simulink model "refrigerationCycle"  (R2014a)
settings: Solver=ode15s  StartTime=0.0  StopTime=3000  MaxStep=0.2  RelTol=1e-3  AbsTol=1e-3
PreLoadFcn:
  | load R134aProperties p_TLU u_TLU v_TLU T_TLU mu_TLU k_TLU Pr_TLU u_sat
  | 
  | % Refrigerant:
  | charge_pressure = 0.6; % MPa
  | initial_quality = 0.2;
  | 
  | % Environment:
  | environment_temperature = 293; % K
  | natural_convection_coefficient = 20; % W/m^2/K
  | 
  | % Controller:
  | target_temperature = 277; % K
  | temperature_delta = 2; % K
  | 
  | % Compressor:
  | commanded_mass_flow = 0.004; % kg/s
  | compressor_time_constant = 20; % s
  | 
  | % Expansion valve:
  | min_throat_area = 0.1; % mm^2
  | max_throat_area = 2.7; % mm^2
  | min_throat_temperature = 280; % K
  | max_throat_temperature = 230; % K
  | 
  | % Heat exchangers:
  | condenser_length = 15; % m
  | evaporator_length = 15; % m
  | fin_area = 1; % m^2
  | fin_convection_coefficient = 150; % W/m^2/K
  | 
  | % Pipes:
  | pipe_diameter = 0.015; % m
  | pipe_thickness = 0.0005; % m
  | 
  | % Refrigerator compartment:
  | interior_surface_area = 4.5; % m^2
  | exterior_surface_area = 6; % m^2
  | foam_thickness = 0.03; % m
  | 
  | % Material properties:
  | copper_density = 8940; % kg/m^3
  | copper_specific_heat = 390; % J/kg/K
  | copper_conductivity = 400; % W/m/K
  | foam_conductivity = 0.03; % W/m/K
undefined symbols (not defined in the file or in its folder): u_sat
libraries: fl_lib x25, refrigeration_lib x19, nesl_utility x5
Description:
  | Two-Phase Flow Refrigeration Model
  | 
  | This example demonstrates a two-phase flow model to simulate a refrigeration cycle.
  | The compressor drives the R-134a refrigerant through a condenser, an expansion valve,
  | and an evaporator. The hot gas leaving the compressor condenses in the condenser via
  | heat transfer to the environment. The pressure drops as the refrigerant passes through
  | the expansion valve. The drop in pressure causes the refrigerant to boil in the evaporator
  | as it absorbs heat from the refrigerator compartment. The refrigeration then returns to
  | the compressor to repeat the cycle. The controller turns the compressor on and off to
  | maintain the refrigerator compartment temperature within a band around the desired
  | temperature.
  | 
  | Copyright 2013-2014 The MathWorks, Inc.
settings Model: Creator=MathWorks  LastModifiedBy=leong
settings SolverCC: MaxConsecutiveMinStep=2
settings DataIOCC: LimitDataPoints=off  SignalLoggingSaveFormat=ModelDataLogs
settings DebuggingCC: MergeDetectMultiDrivingBlocksExec=error  MultiTaskDSMMsg=warning  MultiTaskCondExecSysMsg=none
settings RTWCC: IncludeERTFirstTime=on
settings SimscapeCC: SimscapeLogType=all  SimscapeLogName=refrigerationModelData  SimscapeLogLimitData=off

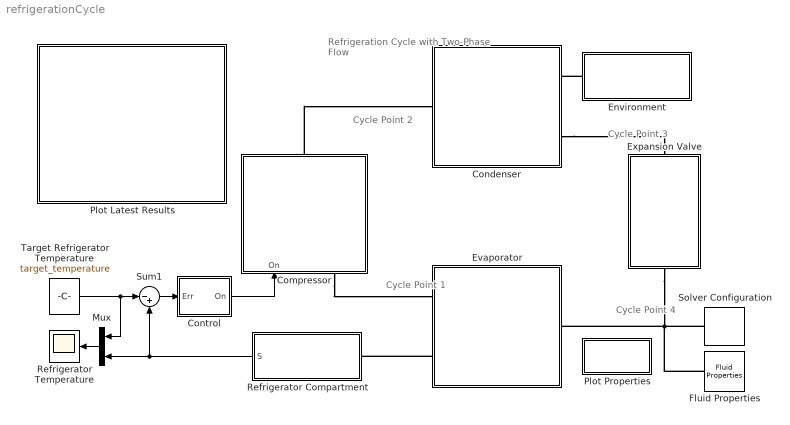
== system refrigerationCycle ==
  note: Cycle Point 1
  note: Cycle Point 2
  note: Cycle Point 3
  note: Refrigeration Cycle
      | with Two-Phase Flow
  note: Cycle Point 4
  Compressor : Subsystem
      mask Display:
      | % Fading color
      | % Center to right
      | patch(sin(0.00*pi:0.05:1.10*pi),cos(0.00*pi:0.05:1.10*pi),[1;0.90;0.94]);
      | patch(sin(0.05*pi:0.05:0.95*pi),cos(0.05*pi:0.05:0.95*pi),[1;0.85;0.88]);
      | patch(sin(0.10*pi:0.05:0.90*pi),cos(0.10*pi:0.05:0.90*pi),[1;0.80;0.82]);
      | patch(sin(0.15*pi:0.05:0.85*pi),cos(0.15*pi:0.05:0.85*pi),[1;0.75;0.76]);
      | patch(sin(0.20*pi:0.05:0.80*pi),cos(0.20*pi:0.05:0.80*pi),[1;0.70;0.70]);
      | % Center to left
      | patch(sin(1.00*pi:0.05:2.00*pi),cos(1.00*pi:0.05:2.00*pi),[0.94;0.90;1]);
      | patch(sin(1.05*pi:0.05:1.95*pi),cos(1.05*pi:0.05:1.95*pi),[0.88;0.90;1]);
      | patch(sin(1.10*pi:0.05:1.90*pi),cos(1.10*pi:0.05:1.90*pi),[0.82;0.90;1]);
      | patch(sin(1.15*pi:0.05:1.85*pi),cos(1.15*pi:0.05:1.85*pi),[0.76;0.90;1]);
      | patch(sin(1.20*pi:0.05:1.80*pi),cos(1.20*pi:0.05:1.80*pi),[0.70;0.90;1]);
      | % Circle
      | plot(sin(0:0.1:2.2*pi),cos(0:0.1:2.2*pi));
      | % Angled lines
      | plot(sin([-0.6*pi/3 3.6*pi/8]),cos([-0.6*pi/3 3.6*pi/8]));
      | plot(sin([-0.6*pi/3 3.6*pi/8]),-cos([-0.6*pi/3 3.6*pi/8]));
      | plot(1.15*sin([-pi/4 3*pi/4]),1.15*cos([-pi/4 3*pi/4]));
      | % Arrow
      | patch([1.15*sin(-pi/4)+0.01;1.15*sin(3*pi/4)+0.01;1.15*sin(3*pi/4)-0.01;1.15*sin(-pi/4)-0.01],[1.15*cos(-pi/4)+0.01;1.15*cos(3*pi/4)+0.01;1.15*cos(3*pi/4)-0.01;1.15*cos(-pi/4)-0.01],[0;0;0])
      | patch([0.8*sin(3*pi/4)+0.05;1.15*sin(3*pi/4)+0.00;1.15*sin(3*pi/4)-0.00;0.8*sin(3*pi/4)-0.05],[0.8*cos(3*pi/4)+0.05;1.15*cos(3*pi/4)+0.00;1.15*cos(3*pi/4)-0.00;0.8*cos(3*pi/4)-0.05],[0;0;0])
      | % Points to set range for plotting area
      | color('white');plot(1.3,1.3);plot(-1.3,-1.3)
      | color('black');
      | 
      | port_label('LConn',1,'A');
      | port_label('RConn',1,'B');
      | port_label('input',1,'On');
  Condenser : Subsystem
      mask Display:
      | % Colored patches
      | % Center to right
      | patch(sin(0.0*pi:0.05:1.1*pi),cos(0.0*pi:0.05:1.1*pi),[1;0.58;0.58]);
      | patch(sin(0.1*pi:0.05:0.9*pi),cos(0.1*pi:0.05:0.9*pi),[1;0.64;0.64]);
      | patch(sin(0.2*pi:0.05:0.8*pi),cos(0.2*pi:0.05:0.8*pi),[1;0.70;0.70]);
      | % Center to left
      | patch(sin(1.0*pi:0.05:2.0*pi),cos(1.0*pi:0.05:2.0*pi),[1;0.52;0.52]);
      | patch(sin(1.1*pi:0.05:1.9*pi),cos(1.1*pi:0.05:1.9*pi),[1;0.46;0.46]);
      | patch(sin(1.2*pi:0.05:1.8*pi),cos(1.2*pi:0.05:1.8*pi),[1;0.40;0.40]);
      | % Circle
      | plot(sin(0:0.1:2.2*pi),cos(0:0.1:2.2*pi));
      | % 'M'
      | plot([0.5 0.5],[-1.2 0.5]);
      | plot([-0.5 -0.5],[-1.2 0.5]);
      | plot([0.5 0],[0.5 -0.2]);
      | plot([-0.5 0],[0.5 -0.2]);
      | % Plot points to set plot range
      | color('white');plot(1.3,1.3);plot(-1.3,-1.3)
      | color('black');
      | 
      | port_label('RConn',1,'A');
      | port_label('LConn',1,'T');
      | port_label('LConn',2,'B');
  Control : Subsystem
  Environment : Subsystem
      mask Display:
      | % Colored patch
      | patch([sin(0:0.1:1*pi)*0.25+0.4 sin(pi:0.1:2*pi)*0.25-0.4],[cos(0:0.1:1*pi) cos(pi:0.1:2*pi)],[1;0.9;0.9]);
      | % Outer rounded rectangle
      | plot(sin(0:0.1:1*pi)*0.25+0.4,cos(0:0.1:1*pi));
      | plot(sin(pi:0.1:2*pi)*0.25-0.4,cos(pi:0.1:2*pi));
      | plot([-0.4 0.4],[1 1]);
      | plot([-0.4 0.4],[-1 -1]);
      | % House frame
      | plot([-0.3 -0.3],[-0.866,0.866*0.2])
      | plot([0.3 0.3],[-0.866,0.866*0.2])
      | plot([0.3 0],[0.866*0.2, 0.866])
      | plot([-0.3 0],[0.866*0.2, 0.866])
      | plot([-0.3 0.3],[-0.866 -0.866])
      | plot([-0.3 0.3],[0.866 0.866]*0.2)
      | plot([-0.2 -0.04],[0.866 0.866]*0)
      | % Window
      | plot([-0.2 -0.04],[-1 -1]*0.2)
      | plot([-0.2 -0.04],[-1 -1]*0.4)
      | plot([-0.2 -0.2],[0 -0.4])
      | plot([-0.12 -0.12],[0 -0.4])
      | plot([-0.04 -0.04],[0 -0.4])
      | % Door
      | plot([0.05 0.05],[-0.866 -0.2])
      | plot([0.18 0.18],[-0.866 -0.2])
      | plot([0.05 0.18],[-0.2 -0.2])
      | patch([0.12 0.15 0.12 0.15],[-0.5 -0.5 -0.54 -0.54],[0;0;0])
      | % Outer boundary (so plot labels are visible)
      | color('white');plot(0.8660,0.8660);plot(-0.8660,-0.8660)
      | color('black');
      | port_label('LConn',1,'T');
  Evaporator : Subsystem
      mask Display:
      | % Fading color
      | % Center to right
      | patch(sin(0.00*pi:0.05:1.10*pi),cos(0.00*pi:0.05:1.10*pi),[0.58;0.70;1]);
      | patch(sin(0.05*pi:0.05:0.95*pi),cos(0.05*pi:0.05:0.95*pi),[0.63;0.75;1]);
      | patch(sin(0.10*pi:0.05:0.90*pi),cos(0.10*pi:0.05:0.90*pi),[0.66;0.80;1]);
      | patch(sin(0.15*pi:0.05:0.85*pi),cos(0.15*pi:0.05:0.85*pi),[0.69;0.85;1]);
      | patch(sin(0.20*pi:0.05:0.80*pi),cos(0.20*pi:0.05:0.80*pi),[0.70;0.90;1]);
      | % Center to left
      | patch(sin(1.00*pi:0.05:2.00*pi),cos(1.00*pi:0.05:2.00*pi),[0.52;0.60;1]);
      | patch(sin(1.05*pi:0.05:1.95*pi),cos(1.05*pi:0.05:1.95*pi),[0.49;0.55;1]);
      | patch(sin(1.10*pi:0.05:1.90*pi),cos(1.10*pi:0.05:1.90*pi),[0.46;0.50;1]);
      | patch(sin(1.15*pi:0.05:1.85*pi),cos(1.15*pi:0.05:1.85*pi),[0.43;0.45;1]);
      | patch(sin(1.20*pi:0.05:1.80*pi),cos(1.20*pi:0.05:1.80*pi),[0.40;0.40;1]);
      | % Circle
      | plot(sin(0:0.1:2.2*pi),cos(0:0.1:2.2*pi));
      | % 'M'
      | plot([0.5 0.5],[-1.2 0.5]);
      | plot([-0.5 -0.5],[-1.2 0.5]);
      | plot([0.5 0],[0.5 -0.2]);
      | plot([-0.5 0],[0.5 -0.2]);
      | % Plot points to set plotting range
      | color('white');plot(1.3,1.3);plot(-1.3,-1.3)
      | color('black');
      | 
      | port_label('LConn',1,'A');
      | port_label('RConn',1,'B');
      | port_label('RConn',2,'T');
  Expansion Valve : Subsystem
      mask Display:
      | % Colored patches
      | patch([-1 -1 0],[0.5 -0.5 0],[1;0.4;0.4]);
      | patch([1 1 0],[0.5 -0.5 0],[0.4;0.4;1]);
      | % Valve
      | plot([1 1],[0.5 -0.5]);
      | plot([-1 -1],[0.5 -0.5]);
      | plot([-1 1],[0.5 -0.5]);
      | plot([-1 1],[-0.5 0.5]);
      | % Arrow
      | patch([1.15*sin(-pi/4-0.01);1.15*sin(-pi/4+0.01);1*sin(3*pi/4-0.01);1*sin(3*pi/4+0.01)],[1.15*cos(-pi/4-0.01);1.15*cos(-pi/4+0.01);1*cos(3*pi/4-0.01);1*cos(3*pi/4+0.01)],[0;0;0])
      | patch([0.8*sin(3*pi/4+0.07);1.15*sin(3*pi/4+0.00);1.15*sin(3*pi/4-0.00);0.8*sin(3*pi/4-0.07)],[0.8*cos(3*pi/4+0.07);1.15*cos(3*pi/4+0.00);1.15*cos(3*pi/4-0.00);0.8*cos(3*pi/4-0.07)],[0;0;0])
      | % Plot outer points to set plot range
      | color('white'); plot(-1.3,0); plot(1.3,0);
      | color('black');
      | port_label('LConn',1,'A');
      | port_label('RConn',1,'B');
  Fluid Properties : refrigeration_lib/Fluid Properties  p_TLU=p_TLU MPa  u_TLU=u_TLU kJ/kg  v_TLU=v_TLU m^3/kg  T_TLU=T_TLU K  mu_TLU=mu_TLU s*uPa  k_TLU=k_TLU W/(m*K)  Pr_TLU=Pr_TLU  u_liq=u_sat(:,1) kJ/kg  u_vap=u_sat(:,2) kJ/kg
  Mux : Mux  Inputs=2
  Plot Latest Results : Subsystem
      settings: OpenFcn=|
      | if exist('refrigerationModelData')
      |    plotRefrigerationModel(refrigerationModelData);
      | else
      |    errordlg('Simulate refrigerationCycle.slx before plotting results');
      | end
      mask Display: image('phDiagram.png')
  Plot Properties : Subsystem
      settings: OpenFcn=plotFluidProperties()
      mask Display: disp('Plot Fluid\nProperties');
  Refrigerator Compartment : Subsystem
      mask Display:
      | % Color
      | patch([sin(0:0.1:1*pi)*0.25+0.4 sin(pi:0.1:2*pi)*0.25-0.4],[cos(0:0.1:1*pi) cos(pi:0.1:2*pi)],[0.70;0.90;1]);
      | % Outer rounded rectangle
      | plot(sin(pi:0.1:2*pi)*0.25-0.4,cos(pi:0.1:2*pi));
      | plot(sin(0:0.1:1*pi)*0.25+0.4,cos(0:0.1:1*pi));
      | plot(sin(pi:0.1:2*pi)*0.25-0.4,cos(pi:0.1:2*pi));
      | plot([-0.4 0.4],[1 1]);
      | plot([-0.4 0.4],[-1 -1]);
      | % Outer points to set size of plot range
      | color('white');plot(0.8660,0.8660);plot(-0.8660,-0.8660)
      | color('black');
      | % Snowflake
      | plot([0 0],[0.8 -0.8]);
      | plot([0 0.1],[0.5 0.7]);
      | plot([0 -0.1],[0.5 0.7]);
      | plot([0 0.1],[-0.5 -0.7]);
      | plot([0 -0.1],[-0.5 -0.7]);
      | plot(0.3*sin([pi/3 4*pi/3]),1*cos([pi/3 4*pi/3]));
      | plot([0.22*sin(pi/3) 0.25*sin(pi/4)],[0.7*cos(pi/3) 0.84*cos(pi/4)]);
      | plot([0.22*sin(pi/3) 0.25*sin(pi/2)],[0.7*cos(pi/3) 0.325*cos(pi/4)]);
      | plot([0.22*sin(pi/3) 0.25*sin(pi/4)],[-0.7*cos(pi/3) -0.84*cos(pi/4)]);
      | plot([0.22*sin(pi/3) 0.25*sin(pi/2)],[-0.7*cos(pi/3) -0.325*cos(pi/4)]);
      | plot(-0.3*sin([pi/3 4*pi/3]),1*cos([pi/3 4*pi/3]));
      | plot([-0.22*sin(pi/3) -0.25*sin(pi/4)],[0.7*cos(pi/3) 0.84*cos(pi/4)]);
      | plot([-0.22*sin(pi/3) -0.25*sin(pi/2)],[0.7*cos(pi/3) 0.325*cos(pi/4)]);
      | plot([-0.22*sin(pi/3) -0.25*sin(pi/4)],[-0.7*cos(pi/3) -0.84*cos(pi/4)]);
      | plot([-0.22*sin(pi/3) -0.25*sin(pi/2)],[-0.7*cos(pi/3) -0.325*cos(pi/4)]);
      | plot([0 0.1],[-0.5 -0.7]);
      | plot([0 -0.1],[-0.5 -0.7]);
      | % Labels
      | port_label('LConn',1,'T');
      | port_label('output',1,'S');
  Refrigerator Temperature : Scope
      settings: TimeRange=3000  YMin=274  YMax=280  SaveName=T
  Solver Configuration : nesl_utility/Solver Configuration  PhysicalDomain=network_engine_domain  SubClassName=solver  LeftPortType=input  RightPortType=generic  Accelerate=off  Tones=[]  Harmonics=[]  SimulateNoise=off  Profile=off  UseLocalSampling=off  EnableSwitchedLinearOptims=on  FrequencyDomain=off  UseCCode=off  RelTol=0.001  AbsTol=1e-06  MinStep=1e-09  ToWorkspace=off  DoDC=off  ResidualTolerance=1e-9  UseLocalSolver=off  LocalSolverChoice=NE_TRAPEZOIDAL_ADVANCER  LocalSolverSampleTime=0.1  DoFixedCost=off  MaxNonlinIter=3  MaxModeIter=2  LinearAlgebra=Sparse  DelaysMemoryBudget=1024  AutomaticFiltering=on  FilteringTimeConstant=0.001
  Sum1 : Sum  Inputs=|-+
  Target Refrigerator Temperature : Constant  Value=target_temperature
  wires:
  Target Refrigerator Temperature/1 -> Sum1/1, Mux/1
  Refrigerator Compartment/1(S) -> Mux/2, Sum1/2
  Sum1/1 -> Control/1(Err)
  Control/1(On) -> Compressor/1(On)
  Mux/1 -> Refrigerator Temperature/1
  connections:
  Solver Configuration/RConn1 -- Fluid Properties/RConn1 -- Evaporator/LConn1 -- Expansion Valve/RConn1
  Compressor/RConn1 -- Condenser/RConn1
  Evaporator/RConn2 -- Refrigerator Compartment/LConn1
  Compressor/LConn1 -- Evaporator/RConn1
  Environment/LConn1 -- Condenser/LConn1
  Condenser/LConn2 -- Expansion Valve/LConn1

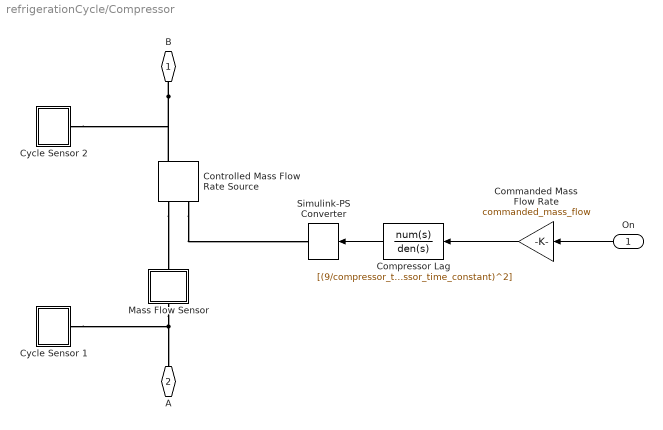
== system refrigerationCycle/Compressor ==
  On : Inport
  Commanded Mass Flow Rate : Gain  Gain=commanded_mass_flow
  Compressor Lag : TransferFcn  Numerator=[(9/compressor_time_constant)^2]  Denominator=[1, 2*(9/compressor_time_constant), (9/compressor_time_constant)^2]
  Controlled Mass Flow Rate Source : refrigeration_lib/Controlled Mass Flow Rate Source  S=pi*pipe_diameter^2/4 m^2  L=0.1 m  mdot_specify=off  mdot_priority=High  mdot=0 kg/s  phi_A_specify=off  phi_A_priority=High  phi_A=0 kW  phi_B_specify=off  phi_B_priority=High  phi_B=0 kW  u_AI_specify=off  u_AI_priority=High  u_AI=396.921741345 kJ/kg  v_A_specify=off  v_A_priority=High  v_A=0.230606289431 m^3/kg  u_BI_specify=off  u_BI_priority=High  u_BI=396.921741345 kJ/kg  v_B_specify=off  v_B_priority=High  v_B=0.230606289431 m^3/kg  u_2_specify=off  u_2_priority=High  u_2=396.921741345 kJ/kg  u_3_specify=off  u_3_priority=High  u_3=396.921741345 kJ/kg
  Cycle Sensor 1 : Subsystem
  Cycle Sensor 2 : Subsystem
  Mass Flow Sensor : Subsystem
  Simulink-PS Converter : nesl_utility/Simulink-PS Converter  PhysicalDomain=network_engine_domain  SubClassName=ps_input  LeftPortType=input  RightPortType=output  PseudoPeriodic=off  Frequencies=[]  NoiseDistribution=none  NoiseParameters=[]  Unit=kg/s  AffineConversion=off  InputFiltering=off  SimscapeFilterOrder=1  InputFilterTimeConstant=0.001  UdotUserProvided=1
  B : PMIOPort  Port=1  Side=Right
  A : PMIOPort  Port=2  Side=Left
  wires:
  Compressor Lag/1 -> Simulink-PS Converter/1
  Commanded Mass Flow Rate/1 -> Compressor Lag/1
  On/1 -> Commanded Mass Flow Rate/1
  connections:
  B/RConn1 -- Cycle Sensor 2/LConn1 -- Controlled Mass Flow Rate Source/RConn1
  Controlled Mass Flow Rate Source/LConn2 -- Simulink-PS Converter/RConn1
  Controlled Mass Flow Rate Source/LConn1 -- Mass Flow Sensor/RConn1
  Mass Flow Sensor/LConn1 -- A/RConn1 -- Cycle Sensor 1/LConn1

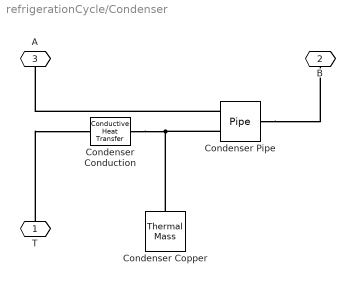
== system refrigerationCycle/Condenser ==
  Condenser Conduction : fl_lib/Thermal/Thermal Elements/Conductive Heat Transfer  area=pi*pipe_diameter*condenser_length m^2  thickness=pipe_thickness m  th_cond=copper_conductivity W/(m*K)  Q_specify=off  Q_priority=High  Q=0 J/s  T_specify=off  T_priority=High  T=0 K
  Condenser Copper : fl_lib/Thermal/Thermal Elements/Thermal Mass  mass=pi*pipe_diameter*condenser_length*pipe_thickness*copper_density kg  sp_heat=copper_specific_heat J/kg/K  Q_specify=off  Q_priority=High  Q=0 J/s  T_specify=on  T_priority=High  T=environment_temperature K
  Condenser Pipe : refrigeration_lib/Pipe  L=condenser_length m  S=pi*pipe_diameter^2/4 m^2  Dh=pipe_diameter m  fs=64  La=0.1*condenser_length m  eps=15e-6 m  Re_lam=2000  Re_tur=4000  J_smooth=5 kg/m^2/s  p_0=charge_pressure MPa  T_0=-1 K  x_0=initial_quality  mdot_A_specify=off  mdot_A_priority=High  mdot_A=0 kg/s  mdot_B_specify=off  mdot_B_priority=High  mdot_B=0 kg/s  phi_A_specify=off  phi_A_priority=High  phi_A=0 kW  phi_B_specify=off  phi_B_priority=High  phi_B=0 kW  v_A_specify=off  v_A_priority=High  v_A=0.230606289431 m^3/kg  v_B_specify=off  v_B_priority=High  v_B=0.230606289431 m^3/kg  p_I_specify=off  p_I_priority=High  p_I=0.101325 MPa  u_I_specify=off  u_I_priority=High  u_I=396.921741345 kJ/kg  v_I_specify=off  v_I_priority=High  v_I=0.230606289431 m^3/kg  q_T_specify=off  q_T_priority=High  q_T=0 kW  Ff_A_specify=off  Ff_A_priority=High  Ff_A=0 N  Ff_B_specify=off  Ff_B_priority=High  Ff_B=0 N  ev_I_specify=off  ev_I_priority=High  ev_I=1.7212095226213e+3 kJ/m^3  mdot_I_specify=off  mdot_I_priority=High  mdot_I=0 kg/s  Nu_I_specify=off  Nu_I_priority=High  Nu_I=0
  T : PMIOPort  Port=1  Side=Left
  B : PMIOPort  Port=2  Side=Left
  A : PMIOPort  Port=3  Side=Right
  connections:
  Condenser Pipe/LConn1 -- A/RConn1
  Condenser Conduction/LConn1 -- Condenser Pipe/LConn2 -- Condenser Copper/LConn1
  T/RConn1 -- Condenser Conduction/RConn1
  Condenser Pipe/RConn1 -- B/RConn1

== system refrigerationCycle/Control ==
  Err : Inport
  Relay : Relay  OnSwitchValue=temperature_delta  OffSwitchValue=-temperature_delta
  On : Outport
  wires:
  Err/1 -> Relay/1
  Relay/1 -> On/1

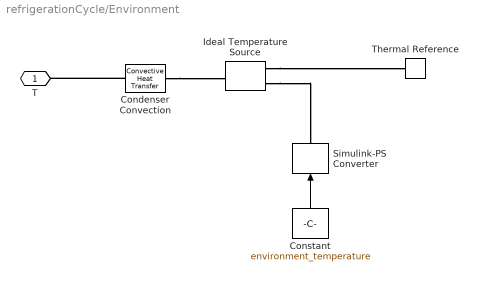
== system refrigerationCycle/Environment ==
  Condenser Convection : fl_lib/Thermal/Thermal Elements/Convective Heat Transfer  area=fin_area m^2  heat_tr_coeff=fin_convection_coefficient W/(m^2 * K)  Q_specify=off  Q_priority=High  Q=0 J/s  T_specify=off  T_priority=High  T=0 K
  Constant : Constant  Value=environment_temperature
  Ideal Temperature Source : fl_lib/Thermal/Thermal Sources/Ideal Temperature Source
  Simulink-PS Converter : nesl_utility/Simulink-PS Converter  PhysicalDomain=network_engine_domain  SubClassName=ps_input  LeftPortType=input  RightPortType=output  PseudoPeriodic=off  Frequencies=[]  NoiseDistribution=none  NoiseParameters=[]  Unit=K  AffineConversion=off  InputFiltering=off  SimscapeFilterOrder=1  InputFilterTimeConstant=0.001  UdotUserProvided=1
  Thermal Reference : fl_lib/Thermal/Thermal Elements/Thermal Reference
  T : PMIOPort  Port=1  Side=Left
  wires:
  Constant/1 -> Simulink-PS Converter/1
  connections:
  Condenser Convection/RConn1 -- Ideal Temperature Source/LConn1
  Condenser Convection/LConn1 -- T/RConn1
  Ideal Temperature Source/RConn1 -- Simulink-PS Converter/RConn1
  Ideal Temperature Source/RConn2 -- Thermal Reference/LConn1

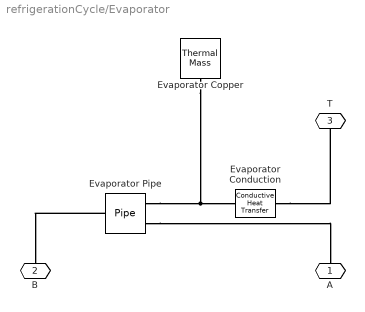
== system refrigerationCycle/Evaporator ==
  Evaporator Conduction : fl_lib/Thermal/Thermal Elements/Conductive Heat Transfer  area=pi*pipe_diameter*evaporator_length m^2  thickness=pipe_thickness m  th_cond=copper_conductivity W/(m*K)  Q_specify=off  Q_priority=High  Q=0 J/s  T_specify=off  T_priority=High  T=0 K
  Evaporator Copper : fl_lib/Thermal/Thermal Elements/Thermal Mass  mass=pi*pipe_diameter*evaporator_length*pipe_thickness*copper_density kg  sp_heat=copper_specific_heat J/kg/K  Q_specify=off  Q_priority=High  Q=0 J/s  T_specify=on  T_priority=High  T=target_temperature K
  Evaporator Pipe : refrigeration_lib/Pipe  L=evaporator_length m  S=pi*pipe_diameter^2/4 m^2  Dh=pipe_diameter m  fs=64  La=0.1*evaporator_length m  eps=15e-6 m  Re_lam=2000  Re_tur=4000  J_smooth=5 kg/m^2/s  p_0=charge_pressure MPa  T_0=-1 K  x_0=initial_quality  mdot_A_specify=off  mdot_A_priority=High  mdot_A=0 kg/s  mdot_B_specify=off  mdot_B_priority=High  mdot_B=0 kg/s  phi_A_specify=off  phi_A_priority=High  phi_A=0 kW  phi_B_specify=off  phi_B_priority=High  phi_B=0 kW  v_A_specify=off  v_A_priority=High  v_A=0.230606289431 m^3/kg  v_B_specify=off  v_B_priority=High  v_B=0.230606289431 m^3/kg  p_I_specify=off  p_I_priority=High  p_I=0.101325 MPa  u_I_specify=off  u_I_priority=High  u_I=396.921741345 kJ/kg  v_I_specify=off  v_I_priority=High  v_I=0.230606289431 m^3/kg  q_T_specify=off  q_T_priority=High  q_T=0 kW  Ff_A_specify=off  Ff_A_priority=High  Ff_A=0 N  Ff_B_specify=off  Ff_B_priority=High  Ff_B=0 N  ev_I_specify=off  ev_I_priority=High  ev_I=1.7212095226213e+3 kJ/m^3  mdot_I_specify=off  mdot_I_priority=High  mdot_I=0 kg/s  Nu_I_specify=off  Nu_I_priority=High  Nu_I=0
  A : PMIOPort  Port=1  Side=Left
  B : PMIOPort  Port=2  Side=Right
  T : PMIOPort  Port=3  Side=Right
  connections:
  Evaporator Conduction/RConn1 -- T/RConn1
  Evaporator Copper/LConn1 -- Evaporator Pipe/LConn2 -- Evaporator Conduction/LConn1
  Evaporator Pipe/RConn1 -- B/RConn1
  Evaporator Pipe/LConn1 -- A/RConn1

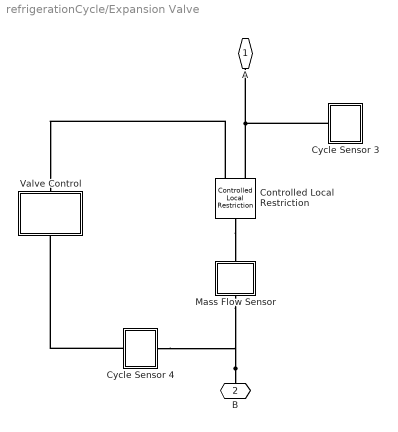
== system refrigerationCycle/Expansion Valve ==
  Controlled Local Restriction : refrigeration_lib/Controlled Local Restriction  Cd=0.7  L=0.1 m  S=pi*pipe_diameter^2/4 m^2
  Cycle Sensor 3 : Subsystem
  Cycle Sensor 4 : Subsystem
  Mass Flow Sensor : Subsystem
  Valve Control : Subsystem
  A : PMIOPort  Port=1  Side=Left
  B : PMIOPort  Port=2  Side=Right
  connections:
  B/RConn1 -- Cycle Sensor 4/LConn1 -- Mass Flow Sensor/RConn1
  Cycle Sensor 3/LConn1 -- Controlled Local Restriction/LConn1 -- A/RConn1
  Controlled Local Restriction/RConn1 -- Mass Flow Sensor/LConn1
  Controlled Local Restriction/LConn2 -- Valve Control/LConn1
  Cycle Sensor 4/RConn1 -- Valve Control/RConn1

== system refrigerationCycle/Plot Latest Results ==

== system refrigerationCycle/Plot Properties ==

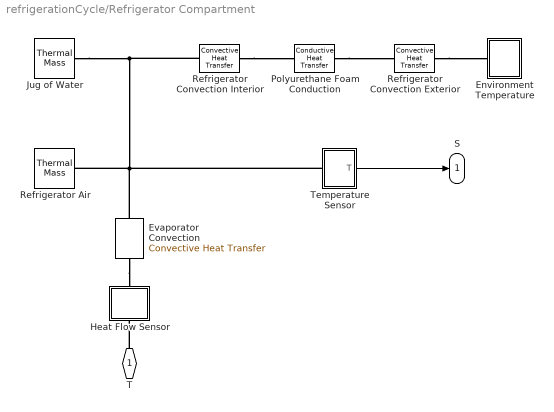
== system refrigerationCycle/Refrigerator Compartment ==
  Environment Temperature : Subsystem
  Evaporator Convection : fl_lib/Thermal/Thermal Elements/Convective Heat Transfer  area=interior_surface_area m^2  heat_tr_coeff=natural_convection_coefficient W/(m^2 * K)  Q_specify=off  Q_priority=High  Q=0 J/s  T_specify=off  T_priority=High  T=0 K
  Heat Flow Sensor : Subsystem
  Jug of Water : fl_lib/Thermal/Thermal Elements/Thermal Mass  mass=3.8 kg  sp_heat=4187 J/kg/K  Q_specify=off  Q_priority=High  Q=0 J/s  T_specify=on  T_priority=High  T=target_temperature K
  Polyurethane Foam Conduction : fl_lib/Thermal/Thermal Elements/Conductive Heat Transfer  area=interior_surface_area m^2  thickness=foam_thickness m  th_cond=foam_conductivity W/(m*K)  Q_specify=off  Q_priority=High  Q=0 J/s  T_specify=off  T_priority=High  T=0 K
  Refrigerator Air : fl_lib/Thermal/Thermal Elements/Thermal Mass  mass=1 kg  sp_heat=1012 J/kg/K  Q_specify=off  Q_priority=High  Q=0 J/s  T_specify=on  T_priority=High  T=target_temperature K
  Refrigerator Convection Exterior : fl_lib/Thermal/Thermal Elements/Convective Heat Transfer  area=exterior_surface_area m^2  heat_tr_coeff=natural_convection_coefficient W/(m^2 * K)  Q_specify=off  Q_priority=High  Q=0 J/s  T_specify=off  T_priority=High  T=0 K
  Refrigerator Convection Interior : fl_lib/Thermal/Thermal Elements/Convective Heat Transfer  area=interior_surface_area m^2  heat_tr_coeff=natural_convection_coefficient W/(m^2 * K)  Q_specify=off  Q_priority=High  Q=0 J/s  T_specify=off  T_priority=High  T=0 K
  Temperature Sensor : Subsystem
  T : PMIOPort  Port=1  Side=Left
  S : Outport
  wires:
  Temperature Sensor/1(T) -> S/1
  connections:
  Evaporator Convection/LConn1 -- Heat Flow Sensor/RConn1
  T/RConn1 -- Heat Flow Sensor/LConn1
  Refrigerator Convection Exterior/RConn1 -- Environment Temperature/LConn1
  Refrigerator Convection Interior/LConn1 -- Jug of Water/LConn1 -- Refrigerator Air/LConn1 -- Temperature Sensor/LConn1 -- Evaporator Convection/RConn1
  Refrigerator Convection Interior/RConn1 -- Polyurethane Foam Conduction/LConn1
  Polyurethane Foam Conduction/RConn1 -- Refrigerator Convection Exterior/LConn1

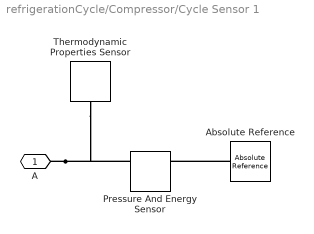
== system refrigerationCycle/Compressor/Cycle Sensor 1 ==
  Absolute Reference : refrigeration_lib/Absolute Reference  mdot_A_specify=off  mdot_A_priority=High  mdot_A=0 kg/s  phi_A_specify=off  phi_A_priority=High  phi_A=0 kW
  Pressure And Energy Sensor : refrigeration_lib/Pressure And Energy Sensor  mdot_specify=off  mdot_priority=High  mdot=0 kg/s  phi_specify=off  phi_priority=High  phi=0 kW
  Thermodynamic Properties Sensor : refrigeration_lib/Thermodynamic Properties Sensor  mdot_A_specify=off  mdot_A_priority=High  mdot_A=0 kg/s  phi_A_specify=off  phi_A_priority=High  phi_A=0 kW
  A : PMIOPort  Port=1  Side=Left
  connections:
  Absolute Reference/LConn1 -- Pressure And Energy Sensor/RConn1
  A/RConn1 -- Thermodynamic Properties Sensor/RConn1 -- Pressure And Energy Sensor/LConn1

== system refrigerationCycle/Compressor/Cycle Sensor 2 ==
  Absolute Reference : refrigeration_lib/Absolute Reference  mdot_A_specify=off  mdot_A_priority=High  mdot_A=0 kg/s  phi_A_specify=off  phi_A_priority=High  phi_A=0 kW
  Pressure And Energy Sensor : refrigeration_lib/Pressure And Energy Sensor  mdot_specify=off  mdot_priority=High  mdot=0 kg/s  phi_specify=off  phi_priority=High  phi=0 kW
  Thermodynamic Properties Sensor : refrigeration_lib/Thermodynamic Properties Sensor  mdot_A_specify=off  mdot_A_priority=High  mdot_A=0 kg/s  phi_A_specify=off  phi_A_priority=High  phi_A=0 kW
  A : PMIOPort  Port=1  Side=Left
  connections:
  Absolute Reference/LConn1 -- Pressure And Energy Sensor/RConn1
  Pressure And Energy Sensor/LConn1 -- A/RConn1 -- Thermodynamic Properties Sensor/RConn1

== system refrigerationCycle/Compressor/Mass Flow Sensor ==
  Mass And Energy Flow Sensor : refrigeration_lib/Mass And Energy Flow Sensor  mdot_specify=off  mdot_priority=High  mdot=0 kg/s  phi_specify=off  phi_priority=High  phi=0 kW
  B : PMIOPort  Port=1  Side=Right
  A : PMIOPort  Port=2  Side=Left
  connections:
  Mass And Energy Flow Sensor/RConn1 -- B/RConn1
  Mass And Energy Flow Sensor/LConn1 -- A/RConn1

== system refrigerationCycle/Expansion Valve/Cycle Sensor 3 ==
  Absolute Reference : refrigeration_lib/Absolute Reference  mdot_A_specify=off  mdot_A_priority=High  mdot_A=0 kg/s  phi_A_specify=off  phi_A_priority=High  phi_A=0 kW
  Pressure And Energy Sensor : refrigeration_lib/Pressure And Energy Sensor  mdot_specify=off  mdot_priority=High  mdot=0 kg/s  phi_specify=off  phi_priority=High  phi=0 kW
  Thermodynamic Properties Sensor : refrigeration_lib/Thermodynamic Properties Sensor  mdot_A_specify=off  mdot_A_priority=High  mdot_A=0 kg/s  phi_A_specify=off  phi_A_priority=High  phi_A=0 kW
  A : PMIOPort  Port=1  Side=Left
  connections:
  Absolute Reference/LConn1 -- Pressure And Energy Sensor/RConn1
  Pressure And Energy Sensor/LConn1 -- A/RConn1 -- Thermodynamic Properties Sensor/RConn1

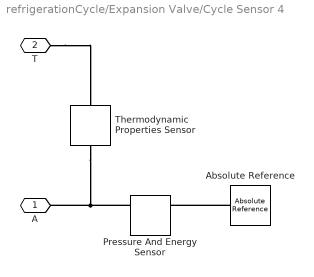
== system refrigerationCycle/Expansion Valve/Cycle Sensor 4 ==
  Absolute Reference : refrigeration_lib/Absolute Reference  mdot_A_specify=off  mdot_A_priority=High  mdot_A=0 kg/s  phi_A_specify=off  phi_A_priority=High  phi_A=0 kW
  Pressure And Energy Sensor : refrigeration_lib/Pressure And Energy Sensor  mdot_specify=off  mdot_priority=High  mdot=0 kg/s  phi_specify=off  phi_priority=High  phi=0 kW
  Thermodynamic Properties Sensor : refrigeration_lib/Thermodynamic Properties Sensor  mdot_A_specify=off  mdot_A_priority=High  mdot_A=0 kg/s  phi_A_specify=off  phi_A_priority=High  phi_A=0 kW
  A : PMIOPort  Port=1  Side=Left
  T : PMIOPort  Port=2  Side=Right
  connections:
  Absolute Reference/LConn1 -- Pressure And Energy Sensor/RConn1
  Pressure And Energy Sensor/LConn1 -- A/RConn1 -- Thermodynamic Properties Sensor/RConn1
  T/RConn1 -- Thermodynamic Properties Sensor/LConn2

== system refrigerationCycle/Expansion Valve/Mass Flow Sensor ==
  Mass And Energy Flow Sensor : refrigeration_lib/Mass And Energy Flow Sensor  mdot_specify=off  mdot_priority=High  mdot=0 kg/s  phi_specify=off  phi_priority=High  phi=0 kW
  B : PMIOPort  Port=1  Side=Right
  A : PMIOPort  Port=2  Side=Left
  connections:
  Mass And Energy Flow Sensor/RConn1 -- B/RConn1
  Mass And Energy Flow Sensor/LConn1 -- A/RConn1

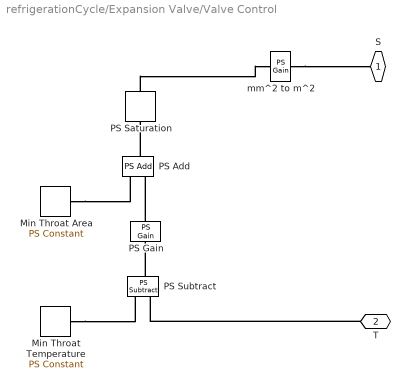
== system refrigerationCycle/Expansion Valve/Valve Control ==
  Min Throat Area : fl_lib/Physical Signals/Sources/PS Constant  constant=min_throat_area
  Min Throat Temperature : fl_lib/Physical Signals/Sources/PS Constant  constant=min_throat_temperature
  PS Add : fl_lib/Physical Signals/Functions/PS Add
  PS Gain : fl_lib/Physical Signals/Functions/PS Gain  gain=(max_throat_area - min_throat_area)/(max_throat_temperature - min_throat_temperature)
  PS Saturation : fl_lib/Physical Signals/Nonlinear Operators/PS Saturation  upper_limit=max_throat_area  lower_limit=min_throat_area
  PS Subtract : fl_lib/Physical Signals/Functions/PS Subtract
  mm^2 to m^2 : fl_lib/Physical Signals/Functions/PS Gain  gain=1e-6
  S : PMIOPort  Port=1  Side=Left
  T : PMIOPort  Port=2  Side=Right
  connections:
  mm^2 to m^2/RConn1 -- S/RConn1
  PS Saturation/RConn1 -- mm^2 to m^2/LConn1
  PS Subtract/RConn1 -- PS Gain/LConn1
  T/RConn1 -- PS Subtract/LConn1
  PS Add/RConn1 -- PS Saturation/LConn1
  Min Throat Area/RConn1 -- PS Add/LConn1
  Min Throat Temperature/RConn1 -- PS Subtract/LConn2
  PS Gain/RConn1 -- PS Add/LConn2

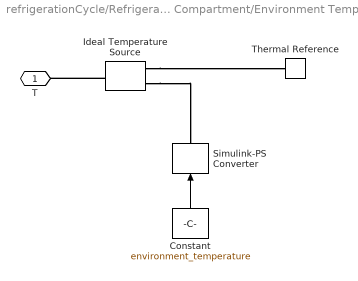
== system refrigerationCycle/Refrigerator Compartment/Environment Temperature ==
  Constant : Constant  Value=environment_temperature
  Ideal Temperature Source : fl_lib/Thermal/Thermal Sources/Ideal Temperature Source
  Simulink-PS Converter : nesl_utility/Simulink-PS Converter  PhysicalDomain=network_engine_domain  SubClassName=ps_input  LeftPortType=input  RightPortType=output  PseudoPeriodic=off  Frequencies=[]  NoiseDistribution=none  NoiseParameters=[]  Unit=K  AffineConversion=off  InputFiltering=off  SimscapeFilterOrder=1  InputFilterTimeConstant=0.001  UdotUserProvided=1
  Thermal Reference : fl_lib/Thermal/Thermal Elements/Thermal Reference
  T : PMIOPort  Port=1  Side=Left
  wires:
  Constant/1 -> Simulink-PS Converter/1
  connections:
  Ideal Temperature Source/RConn2 -- Thermal Reference/LConn1
  Ideal Temperature Source/RConn1 -- Simulink-PS Converter/RConn1
  Ideal Temperature Source/LConn1 -- T/RConn1

== system refrigerationCycle/Refrigerator Compartment/Heat Flow Sensor ==
  Ideal Heat Flow Sensor : fl_lib/Thermal/Thermal Sensors/Ideal Heat Flow Sensor
  B : PMIOPort  Port=1  Side=Right
  A : PMIOPort  Port=2  Side=Left
  connections:
  Ideal Heat Flow Sensor/RConn2 -- B/RConn1
  Ideal Heat Flow Sensor/LConn1 -- A/RConn1

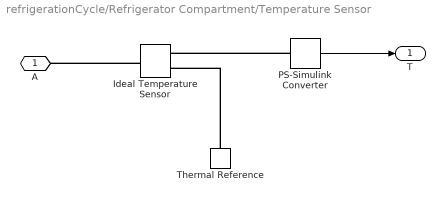
== system refrigerationCycle/Refrigerator Compartment/Temperature Sensor ==
  Ideal Temperature Sensor : fl_lib/Thermal/Thermal Sensors/Ideal Temperature Sensor
  PS-Simulink Converter : nesl_utility/PS-Simulink Converter  PhysicalDomain=network_engine_domain  SubClassName=ps_output  LeftPortType=input  RightPortType=output  PseudoPeriodic=off  Frequencies=[]  Unit=K  AffineConversion=off
  Thermal Reference : fl_lib/Thermal/Thermal Elements/Thermal Reference
  A : PMIOPort  Port=1  Side=Left
  T : Outport
  wires:
  PS-Simulink Converter/1 -> T/1
  connections:
  Ideal Temperature Sensor/LConn1 -- A/RConn1
  Thermal Reference/LConn1 -- Ideal Temperature Sensor/RConn1
  PS-Simulink Converter/LConn1 -- Ideal Temperature Sensor/RConn2
